simulink model "Torrico2019Simu"  (R2018a)
settings: Solver=VariableStepAuto  StartTime=0.0  StopTime=Tsim  RelTol=1e-3
StopFcn:
  | plotSimu
values from neighbouring files (symbols this model uses):
  A = A'    [Bismark2019.m]    (also in Torrico2019.m; Torrico2019Example1.m; Torrico2019Example2.m; Torrico2019Example3.m)
  B = C'    [Bismark2019.m]    (also in Torrico2019.m; Torrico2019Example1.m; Torrico2019Example2.m; Torrico2019Example3.m)
  C = buff    [Bismark2019.m]    (also in Torrico2019.m; Torrico2019Example1.m; Torrico2019Example2.m; Torrico2019Example3.m)
  d = P1z.InputDelay    [Bismark2019.m]    (also in Torrico2019.m; Torrico2019Example1.m; Torrico2019Example2.m; Torrico2019Example3.m)
  K = acker(A,B,beta)    [Bismark2019.m]    (also in Torrico2019.m; Torrico2019Example1.m; Torrico2019Example2.m; Torrico2019Example3.m)
  noiseTime = 55    [Torrico2019Example1.m]    (also in Torrico2019Example2.m = 99; Torrico2019Example3.m = 20)
  Ts = 0.1    [Bismark2019.m]    (also in Torrico2019.m; Torrico2019Example1.m; Torrico2019Example2.m = 0.05; Torrico2019Example3.m = 0.01)
  z = tf('z',Ts)    [Bismark2019.m]    (also in Torrico2019.m; Torrico2019Example1.m; Torrico2019Example2.m; Torrico2019Example3.m)
libraries: cstblocks x5, simulink x1
settings Model: Creator=aluno-2  LastModifiedBy=adriano

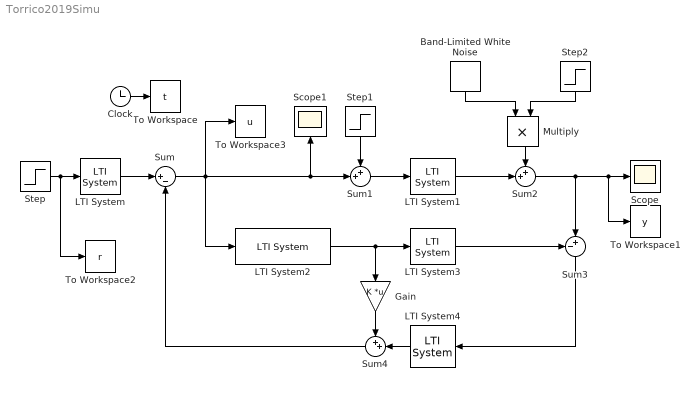
== system Torrico2019Simu ==
  Band-Limited White Noise : simulink/Sources/Band-Limited White Noise  Cov=noisePower  Ts=Ts  seed=[23341]
  Clock : Clock
  Gain : Gain  Gain=K  Multiplication=Matrix(K*u)
  LTI System : cstblocks/LTI System  sys=F  IC=[]
  LTI System1 : cstblocks/LTI System  sys=P1z  IC=[]
  LTI System2 : cstblocks/LTI System  sys=(z*eye(size(A))-A)\B  IC=[]
  LTI System3 : cstblocks/LTI System  sys=C*z^-d  IC=[]
  LTI System4 : cstblocks/LTI System  sys=V  IC=[]
  Multiply : Product
  Scope : Scope
  Scope1 : Scope
  Step : Step  Time=0  SampleTime=0
  Step1 : Step  Time=30  After=-1  SampleTime=0
  Step2 : Step  Time=noiseTime  SampleTime=0
  Sum : Sum  Inputs=|+-
  Sum1 : Sum  Inputs=++|
  Sum2 : Sum  Inputs=++|
  Sum3 : Sum  Inputs=-+|
  Sum4 : Sum  Inputs=++|
  To Workspace : ToWorkspace  VariableName=t  SampleTime=Ts
  To Workspace1 : ToWorkspace  VariableName=y  SampleTime=Ts
  To Workspace2 : ToWorkspace  VariableName=r  SampleTime=Ts
  To Workspace3 : ToWorkspace  VariableName=u  SampleTime=Ts
  wires:
  Step/1 -> To Workspace2/1, LTI System/1
  LTI System/1 -> Sum/1
  Sum1/1 -> LTI System1/1
  LTI System1/1 -> Sum2/2
  Sum4/1 -> Sum/2
  Sum3/1 -> LTI System4/1
  Sum2/1 -> To Workspace1/1, Scope/1, Sum3/2
  LTI System2/1 -> LTI System3/1, Gain/1
  Gain/1 -> Sum4/1
  LTI System3/1 -> Sum3/1
  LTI System4/1 -> Sum4/2
  Step1/1 -> Sum1/1
  Clock/1 -> To Workspace/1
  Sum/1 -> Sum1/2, Scope1/1, LTI System2/1, To Workspace3/1
  Band-Limited White Noise/1 -> Multiply/1
  Step2/1 -> Multiply/2
  Multiply/1 -> Sum2/1
